simulink model "PF"  (R2015a)
settings: Solver=FixedStepDiscrete  SolverMode=SingleTasking  StartTime=0.0  StopTime=2  RelTol=1e-3
libraries: dspsrcs4 x3, dspsnks4 x1, dsparch4 x1
settings Model: DataTypeOverride=Off  Creator=aluno  LastModifiedBy=aluno
settings DataIOCC: SaveOutput=off  SaveTime=off
settings OptimizationCC: BlockReduction=off  ConditionallyExecuteInputs=off  InlineParams=on
settings DebuggingCC: AlgebraicLoopMsg=error  SingleTaskRateTransMsg=error  StrictBusMsg=ErrorOnBusTreatedAsVector
settings HardwareCC: ProdHWDeviceType=ASIC/FPGA->ASIC/FPGA  ProdEqTarget=off

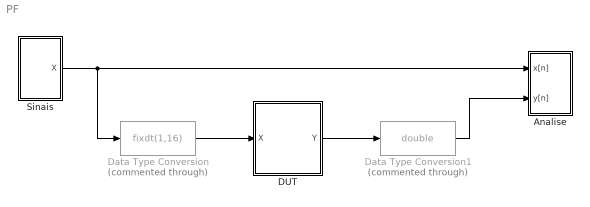
== system PF ==
  Analise : Subsystem
  DUT : Subsystem
  Data Type Conversion : DataTypeConversion  Commented=through  OutMin=-1  OutMax=0.99  OutDataTypeStr=fixdt(1,16)
  Data Type Conversion1 : DataTypeConversion  Commented=through  OutDataTypeStr=double
  Sinais : Subsystem  mask{fa=8000, spf=1, fonte=2, v1=0.5, f1=1000, tchirp=2}
      mask prompts: fa "Freq. amostragem (Hz)"; spf "Amostras por frame"; fonte "Fonte (switch)"; v1 "Amplitude da senoide"; f1 "Freq. da senoide"; tchirp "Tempo Chirp"
      mask TypeOptions fonte: 1 | 2 | 3 | 4 | 5
  wires:
  Sinais/1(X) -> Analise/1(x[n]), Data Type Conversion/1
  Data Type Conversion/1 -> DUT/1(X)
  DUT/1(Y) -> Data Type Conversion1/1
  Data Type Conversion1/1 -> Analise/2(y[n])

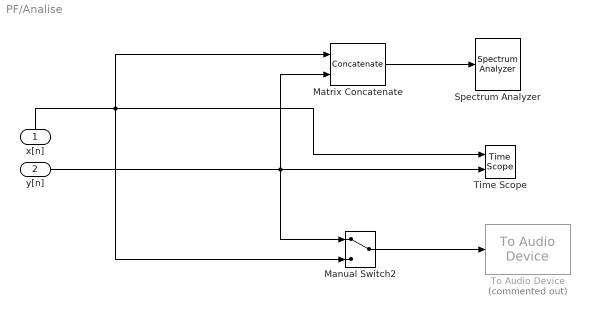
== system PF/Analise ==
  x[n] : Inport
  y[n] : Inport  Port=2
  Manual Switch2 : ManualSwitch
  Matrix Concatenate : Concatenate  Mode=Multidimensional array  ConcatenateDimension=2
  Spectrum Analyzer : SpectrumAnalyzer
  Time Scope : TimeScope  DefaultConfigurationName=spbscopes.TimeScopeBlockCfg  NumInputPorts=2
  To Audio Device : dspsnks4/To Audio Device  Commented=on  deviceName=Default  inheritSampleRate=on  sampleRate=44100  deviceDatatype=Determine from input data type  autoBufferSize=on  bufferSize=4096  queueDuration=1.0  defaultOutputChannelMapping=on  outputChannelMapping=1:2  outputNumUnderrunSamples=off
  wires:
  Matrix Concatenate/1 -> Spectrum Analyzer/1
  x[n]/1 -> Manual Switch2/2, Time Scope/1, Matrix Concatenate/1
  y[n]/1 -> Manual Switch2/1, Matrix Concatenate/2, Time Scope/2
  Manual Switch2/1 -> To Audio Device/1

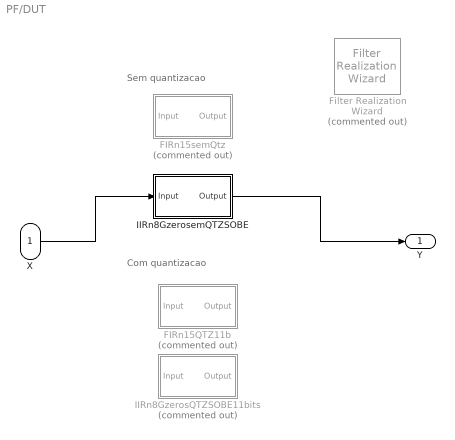
== system PF/DUT ==
  note: Com quantizacao
  note: Sem quantizacao
  X : Inport
  FIRn15QTZ11b : Subsystem  Tag=FilterWizardSubSystem  Commented=on
      settings: ErrorFcn=dspFilterRealizedInBasicElemsAlgLoopErrFcnCallback
  FIRn15semQtz : Subsystem  Tag=FilterWizardSubSystem  Commented=on
      settings: ErrorFcn=dspFilterRealizedInBasicElemsAlgLoopErrFcnCallback
  Filter Realization Wizard : dsparch4/Filter Realization Wizard  Commented=on
  IIRn8GzerosQTZSOBE11bits : Subsystem  Tag=FilterWizardSubSystem  Commented=on
      settings: ErrorFcn=dspFilterRealizedInBasicElemsAlgLoopErrFcnCallback
  IIRn8GzerosemQTZSOBE : Subsystem  Tag=FilterWizardSubSystem
      settings: ErrorFcn=dspFilterRealizedInBasicElemsAlgLoopErrFcnCallback
  Y : Outport
  wires:
  X/1 -> IIRn8GzerosemQTZSOBE/1(Input)
  IIRn8GzerosemQTZSOBE/1(Output) -> Y/1

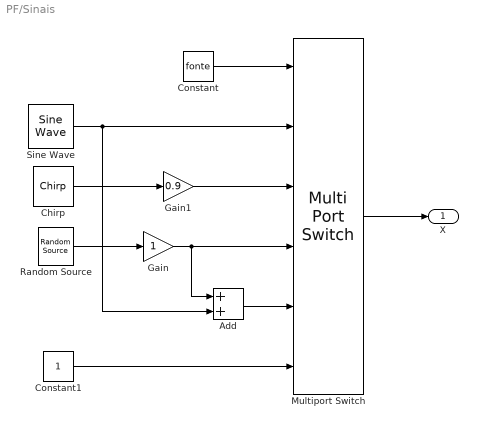
== system PF/Sinais ==
  Add : Sum
  Chirp : dspsrcs4/Chirp  sweep=Linear  mode=Unidirectional  f0=1  f1=fa/2  t1=tchirp  Tsweep=tchirp  phase=0  Ts=1/fa  spf=spf  datatype=Double
  Constant : Constant  Value=fonte
  Constant1 : Constant
  Gain : Gain
  Gain1 : Gain  Gain=0.9
  Multiport Switch : MultiPortSwitch  Inputs=5
  Random Source : dspsrcs4/Random Source  SrcType=Uniform  NormMethod=Ziggurat  CltLength=12  MinVal=-1  MaxVal=1  MeanVal=0  VarVal=1  RepMode=Not repeatable  rawSeed=1  IsInherit=off  SampMode=Discrete  SampTime=1/fa  SampFrame=spf  DataType=Double  OutComplex=Real
  Sine Wave : dspsrcs4/Sine Wave  Amplitude=v1  Frequency=f1  Phase=0  SampleMode=Discrete  OutComplex=Real  CompMethod=Trigonometric fcn  TableSize=Speed  SampleTime=1/fa  SamplesPerFrame=spf  ResetState=Restart at time zero  dataType=double  wordLen=16  udDataType=sfix(16)  fracBitsMode=Best precision  numFracBits=15  OutDataTypeStr=double  LastOutDataTypeStr=double
  X : Outport
  wires:
  Gain/1 -> Add/1, Multiport Switch/4
  Chirp/1 -> Gain1/1
  Sine Wave/1 -> Add/2, Multiport Switch/2
  Multiport Switch/1 -> X/1
  Constant/1 -> Multiport Switch/1
  Add/1 -> Multiport Switch/5
  Constant1/1 -> Multiport Switch/6
  Random Source/1 -> Gain/1
  Gain1/1 -> Multiport Switch/3

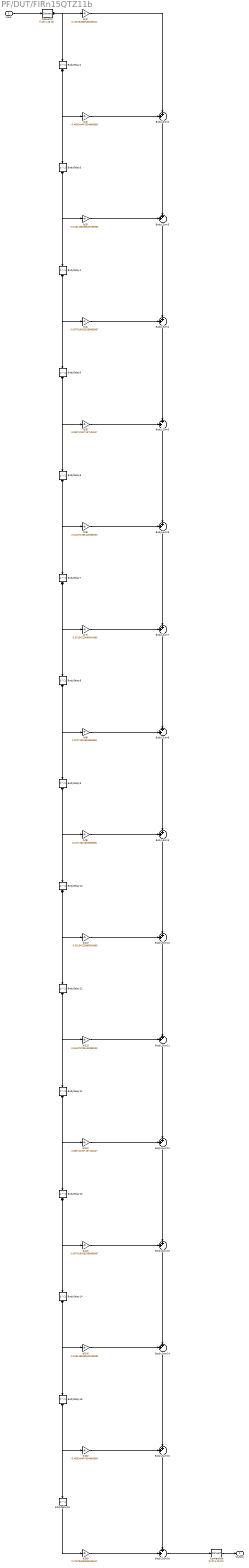
== system PF/DUT/FIRn15QTZ11b ==
  Input : Inport
  BodyDelay{2..16} (15 alike) : Delay  DelayLength=1  InitialCondition=0
  BodyLSum{2..16} (15 alike) : Sum  Inputs=++|  AccumDataTypeStr=fixdt(1,28,23)  OutDataTypeStr=fixdt(1,28,23)  RndMeth=Convergent
  ConvertIn : DataTypeConversion  OutDataTypeStr=fixdt(1,16,15)  RndMeth=Nearest  SaturateOnIntegerOverflow=on
  ConvertOut : DataTypeConversion  OutDataTypeStr=fixdt(1,28,23)  RndMeth=Convergent
  b(1) : Gain  Gain=0.276784850536256011  ParamDataTypeStr=fixdt(1,11,8)  OutDataTypeStr=fixdt(1,26,23)  RndMeth=Convergent
  b(10) : Gain  Gain=-3.30154223899504995  ParamDataTypeStr=fixdt(1,11,8)  OutDataTypeStr=fixdt(1,26,23)  RndMeth=Convergent
  b(11) : Gain  Gain=0.514373785443998033  ParamDataTypeStr=fixdt(1,11,8)  OutDataTypeStr=fixdt(1,26,23)  RndMeth=Convergent
  b(12) : Gain  Gain=0.808711927137104047  ParamDataTypeStr=fixdt(1,11,8)  OutDataTypeStr=fixdt(1,26,23)  RndMeth=Convergent
  b(13) : Gain  Gain=-0.0579194055369869967  ParamDataTypeStr=fixdt(1,11,8)  OutDataTypeStr=fixdt(1,26,23)  RndMeth=Convergent
  b(14) : Gain  Gain=-0.0181458335529195991  ParamDataTypeStr=fixdt(1,11,8)  OutDataTypeStr=fixdt(1,26,23)  RndMeth=Convergent
  b(15) : Gain  Gain=-0.468249447094866988  ParamDataTypeStr=fixdt(1,11,8)  OutDataTypeStr=fixdt(1,26,23)  RndMeth=Convergent
  b(16) : Gain  Gain=0.276784850536256011  ParamDataTypeStr=fixdt(1,11,8)  OutDataTypeStr=fixdt(1,26,23)  RndMeth=Convergent
  b(2) : Gain  Gain=-0.468249447094866988  ParamDataTypeStr=fixdt(1,11,8)  OutDataTypeStr=fixdt(1,26,23)  RndMeth=Convergent
  b(3) : Gain  Gain=-0.0181458335529195991  ParamDataTypeStr=fixdt(1,11,8)  OutDataTypeStr=fixdt(1,26,23)  RndMeth=Convergent
  b(4) : Gain  Gain=-0.0579194055369869967  ParamDataTypeStr=fixdt(1,11,8)  OutDataTypeStr=fixdt(1,26,23)  RndMeth=Convergent
  b(5) : Gain  Gain=0.808711927137104047  ParamDataTypeStr=fixdt(1,11,8)  OutDataTypeStr=fixdt(1,26,23)  RndMeth=Convergent
  b(6) : Gain  Gain=0.514373785443998033  ParamDataTypeStr=fixdt(1,11,8)  OutDataTypeStr=fixdt(1,26,23)  RndMeth=Convergent
  b(7) : Gain  Gain=-3.30154223899504995  ParamDataTypeStr=fixdt(1,11,8)  OutDataTypeStr=fixdt(1,26,23)  RndMeth=Convergent
  b(8) : Gain  Gain=2.20774610833568996  ParamDataTypeStr=fixdt(1,11,8)  OutDataTypeStr=fixdt(1,26,23)  RndMeth=Convergent
  b(9) : Gain  Gain=2.20774610833568996  ParamDataTypeStr=fixdt(1,11,8)  OutDataTypeStr=fixdt(1,26,23)  RndMeth=Convergent
  Output : Outport
  wires:
  Input/1 -> ConvertIn/1
  b(1)/1 -> BodyLSum2/2
  ConvertIn/1 -> b(1)/1, BodyDelay2/1
  BodyDelay2/1 -> b(2)/1, BodyDelay3/1
  b(2)/1 -> BodyLSum2/1
  BodyLSum2/1 -> BodyLSum3/2
  BodyDelay3/1 -> b(3)/1, BodyDelay4/1
  b(3)/1 -> BodyLSum3/1
  BodyLSum3/1 -> BodyLSum4/2
  BodyDelay4/1 -> b(4)/1, BodyDelay5/1
  b(4)/1 -> BodyLSum4/1
  BodyLSum4/1 -> BodyLSum5/2
  BodyDelay5/1 -> b(5)/1, BodyDelay6/1
  b(5)/1 -> BodyLSum5/1
  BodyLSum5/1 -> BodyLSum6/2
  BodyDelay6/1 -> b(6)/1, BodyDelay7/1
  b(6)/1 -> BodyLSum6/1
  BodyLSum6/1 -> BodyLSum7/2
  BodyDelay7/1 -> b(7)/1, BodyDelay8/1
  b(7)/1 -> BodyLSum7/1
  BodyLSum7/1 -> BodyLSum8/2
  BodyDelay8/1 -> b(8)/1, BodyDelay9/1
  b(8)/1 -> BodyLSum8/1
  BodyLSum8/1 -> BodyLSum9/2
  BodyDelay9/1 -> b(9)/1, BodyDelay10/1
  b(9)/1 -> BodyLSum9/1
  BodyLSum9/1 -> BodyLSum10/2
  BodyDelay10/1 -> b(10)/1, BodyDelay11/1
  b(10)/1 -> BodyLSum10/1
  BodyLSum10/1 -> BodyLSum11/2
  BodyDelay11/1 -> b(11)/1, BodyDelay12/1
  b(11)/1 -> BodyLSum11/1
  BodyLSum11/1 -> BodyLSum12/2
  BodyDelay12/1 -> b(12)/1, BodyDelay13/1
  b(12)/1 -> BodyLSum12/1
  BodyLSum12/1 -> BodyLSum13/2
  BodyDelay13/1 -> b(13)/1, BodyDelay14/1
  b(13)/1 -> BodyLSum13/1
  BodyLSum13/1 -> BodyLSum14/2
  BodyDelay14/1 -> b(14)/1, BodyDelay15/1
  b(14)/1 -> BodyLSum14/1
  BodyLSum14/1 -> BodyLSum15/2
  BodyDelay15/1 -> b(15)/1, BodyDelay16/1
  b(15)/1 -> BodyLSum15/1
  BodyLSum15/1 -> BodyLSum16/1
  BodyDelay16/1 -> b(16)/1
  b(16)/1 -> BodyLSum16/2
  BodyLSum16/1 -> ConvertOut/1
  ConvertOut/1 -> Output/1

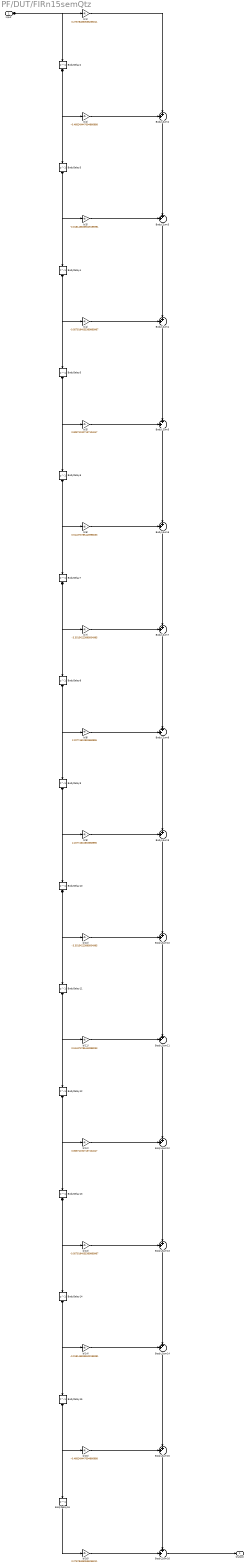
== system PF/DUT/FIRn15semQtz ==
  Input : Inport
  BodyDelay{2..16} (15 alike) : Delay  DelayLength=1  InitialCondition=0  InputProcessing=Columns as channels (frame based)
  BodyLSum{2..16} (15 alike) : Sum  Inputs=++|  RndMeth=Nearest  SaturateOnIntegerOverflow=on  OutDataTypeStr=Inherit: Same as first input
  b(1) : Gain  Gain=0.276784850536256011  ParamDataTypeStr=double  RndMeth=Nearest  SaturateOnIntegerOverflow=on  OutDataTypeStr=Inherit: Same as input
  b(10) : Gain  Gain=-3.30154223899504995  ParamDataTypeStr=double  RndMeth=Nearest  SaturateOnIntegerOverflow=on  OutDataTypeStr=Inherit: Same as input
  b(11) : Gain  Gain=0.514373785443998033  ParamDataTypeStr=double  RndMeth=Nearest  SaturateOnIntegerOverflow=on  OutDataTypeStr=Inherit: Same as input
  b(12) : Gain  Gain=0.808711927137104047  ParamDataTypeStr=double  RndMeth=Nearest  SaturateOnIntegerOverflow=on  OutDataTypeStr=Inherit: Same as input
  b(13) : Gain  Gain=-0.0579194055369869967  ParamDataTypeStr=double  RndMeth=Nearest  SaturateOnIntegerOverflow=on  OutDataTypeStr=Inherit: Same as input
  b(14) : Gain  Gain=-0.0181458335529195991  ParamDataTypeStr=double  RndMeth=Nearest  SaturateOnIntegerOverflow=on  OutDataTypeStr=Inherit: Same as input
  b(15) : Gain  Gain=-0.468249447094866988  ParamDataTypeStr=double  RndMeth=Nearest  SaturateOnIntegerOverflow=on  OutDataTypeStr=Inherit: Same as input
  b(16) : Gain  Gain=0.276784850536256011  ParamDataTypeStr=double  RndMeth=Nearest  SaturateOnIntegerOverflow=on  OutDataTypeStr=Inherit: Same as input
  b(2) : Gain  Gain=-0.468249447094866988  ParamDataTypeStr=double  RndMeth=Nearest  SaturateOnIntegerOverflow=on  OutDataTypeStr=Inherit: Same as input
  b(3) : Gain  Gain=-0.0181458335529195991  ParamDataTypeStr=double  RndMeth=Nearest  SaturateOnIntegerOverflow=on  OutDataTypeStr=Inherit: Same as input
  b(4) : Gain  Gain=-0.0579194055369869967  ParamDataTypeStr=double  RndMeth=Nearest  SaturateOnIntegerOverflow=on  OutDataTypeStr=Inherit: Same as input
  b(5) : Gain  Gain=0.808711927137104047  ParamDataTypeStr=double  RndMeth=Nearest  SaturateOnIntegerOverflow=on  OutDataTypeStr=Inherit: Same as input
  b(6) : Gain  Gain=0.514373785443998033  ParamDataTypeStr=double  RndMeth=Nearest  SaturateOnIntegerOverflow=on  OutDataTypeStr=Inherit: Same as input
  b(7) : Gain  Gain=-3.30154223899504995  ParamDataTypeStr=double  RndMeth=Nearest  SaturateOnIntegerOverflow=on  OutDataTypeStr=Inherit: Same as input
  b(8) : Gain  Gain=2.20774610833568996  ParamDataTypeStr=double  RndMeth=Nearest  SaturateOnIntegerOverflow=on  OutDataTypeStr=Inherit: Same as input
  b(9) : Gain  Gain=2.20774610833568996  ParamDataTypeStr=double  RndMeth=Nearest  SaturateOnIntegerOverflow=on  OutDataTypeStr=Inherit: Same as input
  Output : Outport
  wires:
  Input/1 -> b(1)/1, BodyDelay2/1
  b(1)/1 -> BodyLSum2/2
  BodyDelay2/1 -> b(2)/1, BodyDelay3/1
  b(2)/1 -> BodyLSum2/1
  BodyLSum2/1 -> BodyLSum3/2
  BodyDelay3/1 -> b(3)/1, BodyDelay4/1
  b(3)/1 -> BodyLSum3/1
  BodyLSum3/1 -> BodyLSum4/2
  BodyDelay4/1 -> b(4)/1, BodyDelay5/1
  b(4)/1 -> BodyLSum4/1
  BodyLSum4/1 -> BodyLSum5/2
  BodyDelay5/1 -> b(5)/1, BodyDelay6/1
  b(5)/1 -> BodyLSum5/1
  BodyLSum5/1 -> BodyLSum6/2
  BodyDelay6/1 -> b(6)/1, BodyDelay7/1
  b(6)/1 -> BodyLSum6/1
  BodyLSum6/1 -> BodyLSum7/2
  BodyDelay7/1 -> b(7)/1, BodyDelay8/1
  b(7)/1 -> BodyLSum7/1
  BodyLSum7/1 -> BodyLSum8/2
  BodyDelay8/1 -> b(8)/1, BodyDelay9/1
  b(8)/1 -> BodyLSum8/1
  BodyLSum8/1 -> BodyLSum9/2
  BodyDelay9/1 -> b(9)/1, BodyDelay10/1
  b(9)/1 -> BodyLSum9/1
  BodyLSum9/1 -> BodyLSum10/2
  BodyDelay10/1 -> b(10)/1, BodyDelay11/1
  b(10)/1 -> BodyLSum10/1
  BodyLSum10/1 -> BodyLSum11/2
  BodyDelay11/1 -> b(11)/1, BodyDelay12/1
  b(11)/1 -> BodyLSum11/1
  BodyLSum11/1 -> BodyLSum12/2
  BodyDelay12/1 -> b(12)/1, BodyDelay13/1
  b(12)/1 -> BodyLSum12/1
  BodyLSum12/1 -> BodyLSum13/2
  BodyDelay13/1 -> b(13)/1, BodyDelay14/1
  b(13)/1 -> BodyLSum13/1
  BodyLSum13/1 -> BodyLSum14/2
  BodyDelay14/1 -> b(14)/1, BodyDelay15/1
  b(14)/1 -> BodyLSum14/1
  BodyLSum14/1 -> BodyLSum15/2
  BodyDelay15/1 -> b(15)/1, BodyDelay16/1
  b(15)/1 -> BodyLSum15/1
  BodyLSum15/1 -> BodyLSum16/1
  BodyDelay16/1 -> b(16)/1
  b(16)/1 -> BodyLSum16/2
  BodyLSum16/1 -> Output/1

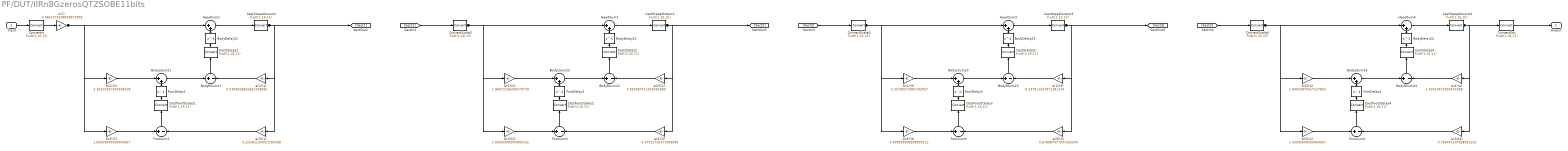
== system PF/DUT/IIRn8GzerosQTZSOBE11bits ==
  Input : Inport
  BodyDelay{21..24} (4 alike) : Delay  DelayLength=1  InitialCondition=0
  BodyLSum{21..24} (4 alike) : Sum  Inputs=|++  AccumDataTypeStr=fixdt(1,40,24)  OutDataTypeStr=fixdt(1,40,24)  RndMeth=Convergent
  BodyRSum{21..24} (4 alike) : Sum  Inputs=+|-  AccumDataTypeStr=fixdt(1,40,24)  OutDataTypeStr=fixdt(1,40,24)  RndMeth=Convergent
  CastFootStates{1..4} (4 alike) : DataTypeConversion  OutDataTypeStr=fixdt(1,16,11)  RndMeth=Convergent
  CastStageOutput{1..4} (4 alike) : DataTypeConversion  OutDataTypeStr=fixdt(1,16,15)  RndMeth=Convergent
  CastStates{1..4} (4 alike) : DataTypeConversion  OutDataTypeStr=fixdt(1,16,11)  RndMeth=Convergent
  ConvertIn : DataTypeConversion  OutDataTypeStr=fixdt(1,16,15)  RndMeth=Nearest  SaturateOnIntegerOverflow=on
  ConvertOut : DataTypeConversion  OutDataTypeStr=fixdt(1,16,11)  RndMeth=Convergent
  ConvertScale2 : DataTypeConversion  OutDataTypeStr=fixdt(1,16,15)  RndMeth=Convergent
  ConvertScale3 : DataTypeConversion  OutDataTypeStr=fixdt(1,16,15)  RndMeth=Convergent
  ConvertScale4 : DataTypeConversion  OutDataTypeStr=fixdt(1,16,15)  RndMeth=Convergent
  FootDelay{1..4} (4 alike) : Delay  DelayLength=1  InitialCondition=0
  FootSum{1..4} (4 alike) : Sum  Inputs=+|-  AccumDataTypeStr=fixdt(1,40,24)  OutDataTypeStr=fixdt(1,40,24)  RndMeth=Convergent
  HeadSum{1..4} (4 alike) : Sum  Inputs=|++  AccumDataTypeStr=fixdt(1,40,24)  OutDataTypeStr=fixdt(1,40,24)  RndMeth=Convergent
  a(2)(1) : Gain  Gain=0.0360556855663169695  ParamDataTypeStr=fixdt(1,11,9)  OutDataTypeStr=fixdt(1,27,24)  RndMeth=Convergent
  a(2)(2) : Gain  Gain=0.950387411024563589  ParamDataTypeStr=fixdt(1,11,9)  OutDataTypeStr=fixdt(1,27,24)  RndMeth=Convergent
  a(2)(3) : Gain  Gain=-0.297811507871281134  ParamDataTypeStr=fixdt(1,11,9)  OutDataTypeStr=fixdt(1,27,24)  RndMeth=Convergent
  a(2)(4) : Gain  Gain=1.40320475024572588  ParamDataTypeStr=fixdt(1,11,9)  OutDataTypeStr=fixdt(1,27,24)  RndMeth=Convergent
  a(3)(1) : Gain  Gain=0.225452234913183308  ParamDataTypeStr=fixdt(1,11,9)  OutDataTypeStr=fixdt(1,27,24)  RndMeth=Convergent
  a(3)(2) : Gain  Gain=0.37322742377099094  ParamDataTypeStr=fixdt(1,11,9)  OutDataTypeStr=fixdt(1,27,24)  RndMeth=Convergent
  a(3)(3) : Gain  Gain=0.678887977937353004  ParamDataTypeStr=fixdt(1,11,9)  OutDataTypeStr=fixdt(1,27,24)  RndMeth=Convergent
  a(3)(4) : Gain  Gain=0.785441107698052532  ParamDataTypeStr=fixdt(1,11,9)  OutDataTypeStr=fixdt(1,27,24)  RndMeth=Convergent
  b(2)(1) : Gain  Gain=-1.82432917633608138  ParamDataTypeStr=fixdt(1,11,9)  OutDataTypeStr=fixdt(1,27,24)  RndMeth=Convergent
  b(2)(2) : Gain  Gain=1.96872166390579739  ParamDataTypeStr=fixdt(1,11,9)  OutDataTypeStr=fixdt(1,27,24)  RndMeth=Convergent
  b(2)(3) : Gain  Gain=-1.25700572885782957  ParamDataTypeStr=fixdt(1,11,9)  OutDataTypeStr=fixdt(1,27,24)  RndMeth=Convergent
  b(2)(4) : Gain  Gain=1.84933870417127855  ParamDataTypeStr=fixdt(1,11,9)  OutDataTypeStr=fixdt(1,27,24)  RndMeth=Convergent
  b(3)(1) : Gain  Gain=1.00000000000000067  ParamDataTypeStr=fixdt(1,11,9)  OutDataTypeStr=fixdt(1,27,24)  RndMeth=Convergent
  b(3)(2) : Gain  Gain=1.00000000000000155  ParamDataTypeStr=fixdt(1,11,9)  OutDataTypeStr=fixdt(1,27,24)  RndMeth=Convergent
  b(3)(3) : Gain  Gain=0.999999999999999112  ParamDataTypeStr=fixdt(1,11,9)  OutDataTypeStr=fixdt(1,27,24)  RndMeth=Convergent
  b(3)(4) : Gain  Gain=1.00000000000000067  ParamDataTypeStr=fixdt(1,11,9)  OutDataTypeStr=fixdt(1,27,24)  RndMeth=Convergent
  s(1) : Gain  Gain=0.0647375508078679995  ParamDataTypeStr=fixdt(1,11,13)  OutDataTypeStr=fixdt(1,16,15)  RndMeth=Convergent
  Output : Outport
  wires:
  Input/1 -> ConvertIn/1
  s(1)/1 -> HeadSum1/1, b(2)(1)/1, b(3)(1)/1
  HeadSum1/1 -> CastStageOutput1/1
  CastStageOutput1/1 -> [Sect1], a(2)(1)/1, a(3)(1)/1
  b(2)(1)/1 -> BodyLSum21/1
  BodyLSum21/1 -> BodyRSum21/1
  BodyRSum21/1 -> CastStates1/1
  a(2)(1)/1 -> BodyRSum21/2
  BodyDelay21/1 -> HeadSum1/2
  b(3)(1)/1 -> FootSum1/1
  FootSum1/1 -> CastFootStates1/1
  a(3)(1)/1 -> FootSum1/2
  FootDelay1/1 -> BodyLSum21/2
  ConvertIn/1 -> s(1)/1
  CastStates1/1 -> BodyDelay21/1
  CastFootStates1/1 -> FootDelay1/1
  [Sect1] -> ConvertScale2/1
  ConvertScale2/1 -> HeadSum2/1, b(2)(2)/1, b(3)(2)/1
  HeadSum2/1 -> CastStageOutput2/1
  CastStageOutput2/1 -> [Sect2], a(2)(2)/1, a(3)(2)/1
  b(2)(2)/1 -> BodyLSum22/1
  BodyLSum22/1 -> BodyRSum22/1
  BodyRSum22/1 -> CastStates2/1
  a(2)(2)/1 -> BodyRSum22/2
  BodyDelay22/1 -> HeadSum2/2
  b(3)(2)/1 -> FootSum2/1
  FootSum2/1 -> CastFootStates2/1
  a(3)(2)/1 -> FootSum2/2
  FootDelay2/1 -> BodyLSum22/2
  CastStates2/1 -> BodyDelay22/1
  CastFootStates2/1 -> FootDelay2/1
  [Sect2] -> ConvertScale3/1
  ConvertScale3/1 -> HeadSum3/1, b(2)(3)/1, b(3)(3)/1
  HeadSum3/1 -> CastStageOutput3/1
  CastStageOutput3/1 -> [Sect3], a(2)(3)/1, a(3)(3)/1
  b(2)(3)/1 -> BodyLSum23/1
  BodyLSum23/1 -> BodyRSum23/1
  BodyRSum23/1 -> CastStates3/1
  a(2)(3)/1 -> BodyRSum23/2
  BodyDelay23/1 -> HeadSum3/2
  b(3)(3)/1 -> FootSum3/1
  FootSum3/1 -> CastFootStates3/1
  a(3)(3)/1 -> FootSum3/2
  FootDelay3/1 -> BodyLSum23/2
  CastStates3/1 -> BodyDelay23/1
  CastFootStates3/1 -> FootDelay3/1
  [Sect3] -> ConvertScale4/1
  ConvertScale4/1 -> HeadSum4/1, b(2)(4)/1, b(3)(4)/1
  HeadSum4/1 -> CastStageOutput4/1
  CastStageOutput4/1 -> ConvertOut/1, a(2)(4)/1, a(3)(4)/1
  b(2)(4)/1 -> BodyLSum24/1
  BodyLSum24/1 -> BodyRSum24/1
  BodyRSum24/1 -> CastStates4/1
  a(2)(4)/1 -> BodyRSum24/2
  BodyDelay24/1 -> HeadSum4/2
  b(3)(4)/1 -> FootSum4/1
  FootSum4/1 -> CastFootStates4/1
  a(3)(4)/1 -> FootSum4/2
  FootDelay4/1 -> BodyLSum24/2
  ConvertOut/1 -> Output/1
  CastStates4/1 -> BodyDelay24/1
  CastFootStates4/1 -> FootDelay4/1

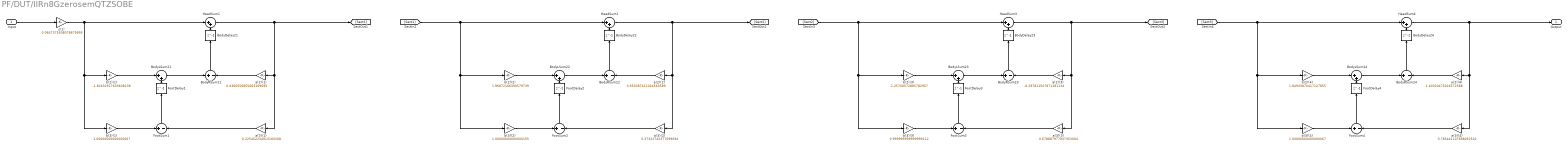
== system PF/DUT/IIRn8GzerosemQTZSOBE ==
  Input : Inport
  BodyDelay{21..24} (4 alike) : Delay  DelayLength=1  InitialCondition=0
  BodyLSum{21..24} (4 alike) : Sum  Inputs=|++  RndMeth=Nearest  SaturateOnIntegerOverflow=on  OutDataTypeStr=Inherit: Same as first input
  BodyRSum{21..24} (4 alike) : Sum  Inputs=+|-  RndMeth=Nearest  SaturateOnIntegerOverflow=on  OutDataTypeStr=Inherit: Same as first input
  FootDelay{1..4} (4 alike) : Delay  DelayLength=1  InitialCondition=0
  FootSum{1..4} (4 alike) : Sum  Inputs=+|-  RndMeth=Nearest  SaturateOnIntegerOverflow=on  OutDataTypeStr=Inherit: Same as first input
  HeadSum{1..4} (4 alike) : Sum  Inputs=|++  RndMeth=Nearest  SaturateOnIntegerOverflow=on  OutDataTypeStr=Inherit: Same as first input
  a(2)(1) : Gain  Gain=0.0360556855663169695  ParamDataTypeStr=double  RndMeth=Nearest  SaturateOnIntegerOverflow=on  OutDataTypeStr=Inherit: Same as input
  a(2)(2) : Gain  Gain=0.950387411024563589  ParamDataTypeStr=double  RndMeth=Nearest  SaturateOnIntegerOverflow=on  OutDataTypeStr=Inherit: Same as input
  a(2)(3) : Gain  Gain=-0.297811507871281134  ParamDataTypeStr=double  RndMeth=Nearest  SaturateOnIntegerOverflow=on  OutDataTypeStr=Inherit: Same as input
  a(2)(4) : Gain  Gain=1.40320475024572588  ParamDataTypeStr=double  RndMeth=Nearest  SaturateOnIntegerOverflow=on  OutDataTypeStr=Inherit: Same as input
  a(3)(1) : Gain  Gain=0.225452234913183308  ParamDataTypeStr=double  RndMeth=Nearest  SaturateOnIntegerOverflow=on  OutDataTypeStr=Inherit: Same as input
  a(3)(2) : Gain  Gain=0.37322742377099094  ParamDataTypeStr=double  RndMeth=Nearest  SaturateOnIntegerOverflow=on  OutDataTypeStr=Inherit: Same as input
  a(3)(3) : Gain  Gain=0.678887977937353004  ParamDataTypeStr=double  RndMeth=Nearest  SaturateOnIntegerOverflow=on  OutDataTypeStr=Inherit: Same as input
  a(3)(4) : Gain  Gain=0.785441107698052532  ParamDataTypeStr=double  RndMeth=Nearest  SaturateOnIntegerOverflow=on  OutDataTypeStr=Inherit: Same as input
  b(2)(1) : Gain  Gain=-1.82432917633608138  ParamDataTypeStr=double  RndMeth=Nearest  SaturateOnIntegerOverflow=on  OutDataTypeStr=Inherit: Same as input
  b(2)(2) : Gain  Gain=1.96872166390579739  ParamDataTypeStr=double  RndMeth=Nearest  SaturateOnIntegerOverflow=on  OutDataTypeStr=Inherit: Same as input
  b(2)(3) : Gain  Gain=-1.25700572885782957  ParamDataTypeStr=double  RndMeth=Nearest  SaturateOnIntegerOverflow=on  OutDataTypeStr=Inherit: Same as input
  b(2)(4) : Gain  Gain=1.84933870417127855  ParamDataTypeStr=double  RndMeth=Nearest  SaturateOnIntegerOverflow=on  OutDataTypeStr=Inherit: Same as input
  b(3)(1) : Gain  Gain=1.00000000000000067  ParamDataTypeStr=double  RndMeth=Nearest  SaturateOnIntegerOverflow=on  OutDataTypeStr=Inherit: Same as input
  b(3)(2) : Gain  Gain=1.00000000000000155  ParamDataTypeStr=double  RndMeth=Nearest  SaturateOnIntegerOverflow=on  OutDataTypeStr=Inherit: Same as input
  b(3)(3) : Gain  Gain=0.999999999999999112  ParamDataTypeStr=double  RndMeth=Nearest  SaturateOnIntegerOverflow=on  OutDataTypeStr=Inherit: Same as input
  b(3)(4) : Gain  Gain=1.00000000000000067  ParamDataTypeStr=double  RndMeth=Nearest  SaturateOnIntegerOverflow=on  OutDataTypeStr=Inherit: Same as input
  s(1) : Gain  Gain=0.0647375508078679995  ParamDataTypeStr=double  RndMeth=Nearest  SaturateOnIntegerOverflow=on  OutDataTypeStr=Inherit: Same as input
  Output : Outport
  wires:
  Input/1 -> s(1)/1
  s(1)/1 -> b(2)(1)/1, b(3)(1)/1, HeadSum1/1
  HeadSum1/1 -> a(2)(1)/1, a(3)(1)/1, [Sect1]
  b(2)(1)/1 -> BodyLSum21/1
  BodyLSum21/1 -> BodyRSum21/1
  BodyRSum21/1 -> BodyDelay21/1
  a(2)(1)/1 -> BodyRSum21/2
  BodyDelay21/1 -> HeadSum1/2
  b(3)(1)/1 -> FootSum1/1
  FootSum1/1 -> FootDelay1/1
  a(3)(1)/1 -> FootSum1/2
  FootDelay1/1 -> BodyLSum21/2
  [Sect1] -> b(2)(2)/1, b(3)(2)/1, HeadSum2/1
  HeadSum2/1 -> a(2)(2)/1, a(3)(2)/1, [Sect2]
  b(2)(2)/1 -> BodyLSum22/1
  BodyLSum22/1 -> BodyRSum22/1
  BodyRSum22/1 -> BodyDelay22/1
  a(2)(2)/1 -> BodyRSum22/2
  BodyDelay22/1 -> HeadSum2/2
  b(3)(2)/1 -> FootSum2/1
  FootSum2/1 -> FootDelay2/1
  a(3)(2)/1 -> FootSum2/2
  FootDelay2/1 -> BodyLSum22/2
  [Sect2] -> b(2)(3)/1, b(3)(3)/1, HeadSum3/1
  HeadSum3/1 -> a(2)(3)/1, a(3)(3)/1, [Sect3]
  b(2)(3)/1 -> BodyLSum23/1
  BodyLSum23/1 -> BodyRSum23/1
  BodyRSum23/1 -> BodyDelay23/1
  a(2)(3)/1 -> BodyRSum23/2
  BodyDelay23/1 -> HeadSum3/2
  b(3)(3)/1 -> FootSum3/1
  FootSum3/1 -> FootDelay3/1
  a(3)(3)/1 -> FootSum3/2
  FootDelay3/1 -> BodyLSum23/2
  [Sect3] -> b(2)(4)/1, b(3)(4)/1, HeadSum4/1
  HeadSum4/1 -> a(2)(4)/1, a(3)(4)/1, Output/1
  b(2)(4)/1 -> BodyLSum24/1
  BodyLSum24/1 -> BodyRSum24/1
  BodyRSum24/1 -> BodyDelay24/1
  a(2)(4)/1 -> BodyRSum24/2
  BodyDelay24/1 -> HeadSum4/2
  b(3)(4)/1 -> FootSum4/1
  FootSum4/1 -> FootDelay4/1
  a(3)(4)/1 -> FootSum4/2
  FootDelay4/1 -> BodyLSum24/2
